simulink model "simulacion"  (R2018a)
settings: Solver=FixedStepAuto  StartTime=0.0  StopTime=20  FixedStep=T/10  RelTol=1e-3
values from neighbouring files (symbols this model uses):
  A = modelo3var.A    [caso.m]    (also in caso2.m; regulador.m = kron(eye(horizon),[1;-1]))
  B = modelo3var.B    [caso.m]    (also in caso2.m; regulador.m = zeros(horizon*m,horizon*n))
  C = modelo3var.C    [caso.m]    (also in caso2.m; prueba.m = 0.5; regulador.m = sysd.C)
  K = [KK(1) KK(2) KK(3)]    [caso2.m]    (also in prueba.m)
  KI = -KK(4)    [caso2.m]    (also in prueba.m)
  T = 0.01    [caso2.m]    (also in prueba.m = 0.05)
libraries: simulink x1
settings Model: Creator=carma  LastModifiedBy=carma

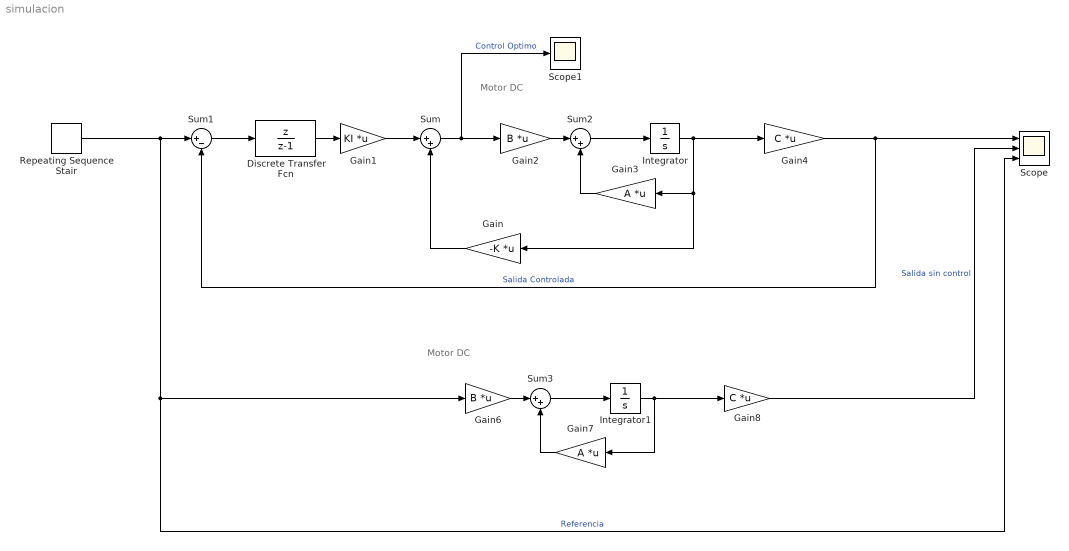
== system simulacion ==
  note: Motor DC
  note: Motor DC
  Discrete Transfer Fcn : DiscreteTransferFcn  Numerator=[1 0]  Denominator=[1 -1]  SampleTime=T
  Gain : Gain  Gain=-K  Multiplication=Matrix(K*u)
  Gain1 : Gain  Gain=KI  Multiplication=Matrix(K*u)
  Gain2 : Gain  Gain=B  Multiplication=Matrix(K*u)
  Gain3 : Gain  Gain=A  Multiplication=Matrix(K*u)
  Gain4 : Gain  Gain=C  Multiplication=Matrix(K*u)
  Gain6 : Gain  Gain=B  Multiplication=Matrix(K*u)
  Gain7 : Gain  Gain=A  Multiplication=Matrix(K*u)
  Gain8 : Gain  Gain=C  Multiplication=Matrix(K*u)
  Integrator : Integrator
  Integrator1 : Integrator
  Repeating Sequence Stair : simulink/Sources/Repeating Sequence Stair  OutValues=[3 -1 4 -2 1].'  tsamp=7  OutMin=[]  OutMax=[]  OutDataTypeStr=double  OutputDataTypeScalingMode=double  OutDataType=fixdt(0,8)  ConRadixGroup=Best Precision: Vector-wise  OutScaling=2^-12
  Scope : Scope  NumInputPorts=3
  Scope1 : Scope
  Sum : Sum  Inputs=|++
  Sum1 : Sum  Inputs=|+-
  Sum2 : Sum  Inputs=|++
  Sum3 : Sum  Inputs=|++
  wires:
  Sum/1 -> Scope1/1, Gain2/1  "Control Optimo"
  Gain/1 -> Sum/2
  Gain4/1 -> Scope/1, Sum1/2  "Salida Controlada"
  Gain1/1 -> Sum/1
  Gain2/1 -> Sum2/1
  Gain3/1 -> Sum2/2
  Sum2/1 -> Integrator/1
  Integrator/1 -> Gain4/1, Gain3/1, Gain/1
  Sum3/1 -> Integrator1/1
  Integrator1/1 -> Gain8/1, Gain7/1
  Gain7/1 -> Sum3/2
  Gain6/1 -> Sum3/1
  Gain8/1 -> Scope/2  "Salida sin control"
  Repeating Sequence Stair/1 -> Scope/3, Gain6/1, Sum1/1  "Referencia"
  Sum1/1 -> Discrete Transfer Fcn/1
  Discrete Transfer Fcn/1 -> Gain1/1
